simulink model "WhippleModel_cont"  (R2018a)
settings: Solver=VariableStepAuto  StartTime=0.0  StopTime=7  MaxStep=0.01  RelTol=1e-3
values from neighbouring files (symbols this model uses):
  sys_Whipple_cont = ss(A,B,C,D)    [DynamicModelParameters.m]
libraries: simulink_extras x2, simulink x1
settings Model: Creator=ProjectHT2018-2  LastModifiedBy=Tom
settings DebuggingCC: LibraryContextMissingDiagnostic=warning
settings SFSimCC: SimUseLocalCustomCode=on
settings RTWCC: RTWUseLocalCustomCode=on

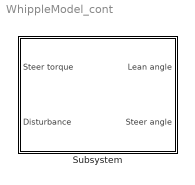
== system WhippleModel_cont ==
  Subsystem : Subsystem

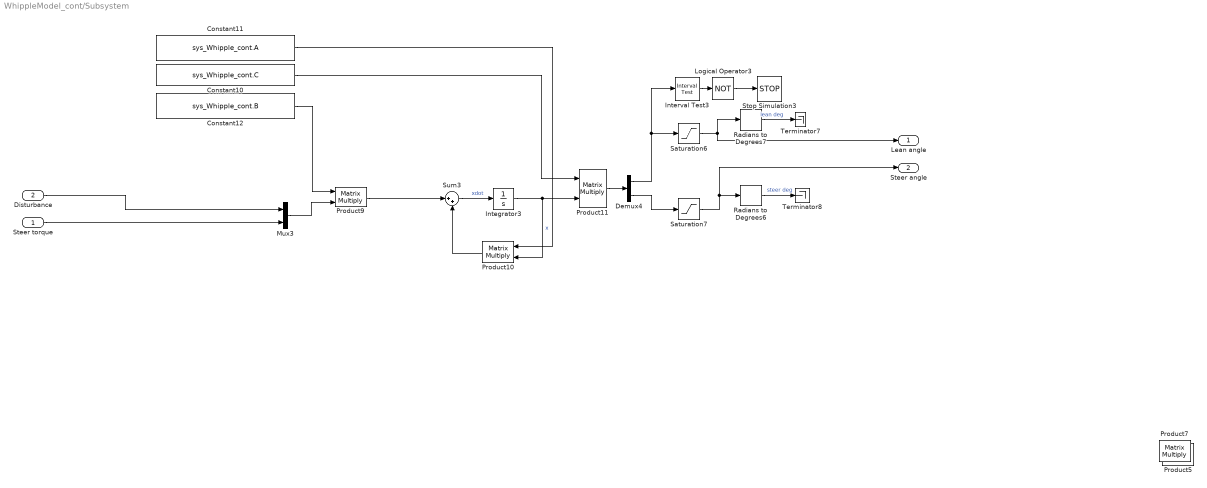
== system WhippleModel_cont/Subsystem ==
  Steer torque : Inport
  Disturbance : Inport  Port=2
  Constant10 : Constant  Value=sys_Whipple_cont.C
  Constant11 : Constant  Value=sys_Whipple_cont.A
  Constant12 : Constant  Value=sys_Whipple_cont.B
  Demux4 : Demux  Outputs=2
  Integrator3 : Integrator
  Interval Test3 : simulink/Logic and Bit Operations/Interval Test  IntervalClosedRight=on  uplimit=pi/4  IntervalClosedLeft=on  lowlimit=-pi/4  OutDataTypeStr=boolean
  Logical Operator3 : Logic  Operator=NOT  AllPortsSameDT=off  OutDataTypeStr=boolean
  Mux3 : Mux  Inputs=2
  Product{5,7,9..11} (5 alike) : Product  Multiplication=Matrix(*)
  Radians to Degrees6 : simulink_extras/Transformations/Radians to Degrees
  Radians to Degrees7 : simulink_extras/Transformations/Radians to Degrees
  Saturation6 : Saturate  UpperLimit=pi/2  LowerLimit=-pi/2
  Saturation7 : Saturate  UpperLimit=pi/2  LowerLimit=-pi/2
  Stop Simulation3 : Stop
  Sum3 : Sum  Inputs=|++
  Terminator7 : Terminator
  Terminator8 : Terminator
  "Lean angle " : Outport
  Steer angle : Outport  Port=2
  wires:
  Constant10/1 -> Product11/1
  Mux3/1 -> Product9/2
  Disturbance/1 -> Mux3/1
  Product9/1 -> Sum3/1
  Steer torque/1 -> Mux3/2
  Demux4/2 -> Saturation7/1
  Constant12/1 -> Product9/1
  Saturation7/1 -> Steer angle/1, Radians to Degrees6/1
  Interval Test3/1 -> Logical Operator3/1
  Sum3/1 -> Integrator3/1  "xdot"
  Radians to Degrees6/1 -> Terminator8/1  "steer deg"
  Saturation6/1 -> "Lean angle "/1, Radians to Degrees7/1
  Demux4/1 -> Interval Test3/1, Saturation6/1
  Product11/1 -> Demux4/1
  Integrator3/1 -> Product10/2, Product11/2  "x"
  Product10/1 -> Sum3/2
  Constant11/1 -> Product10/1
  Logical Operator3/1 -> Stop Simulation3/1
  Radians to Degrees7/1 -> Terminator7/1  "lean deg"
